simulink model "ControllerDesignModel_2023a"  (R2023a)
settings: Solver=FixedStepAuto  StartTime=0.0  StopTime=10  FixedStep=1/1000  RelTol=1e-3
values from neighbouring files (symbols this model uses):
  A = [-2.10   375 ... (first row only)    [ControllerDesign.m]
  B = [ 77 ... (first row only)    [ControllerDesign.m]
  C = [1 0 ... (first row only)    [ControllerDesign.m]
  D = [ 0 ... (first row only)    [ControllerDesign.m]
  IC = [0 deg2rad(30)]    [ControllerDesign.m]
  Kq = 0.17    [ControllerDesign.m]
libraries: simulink_extras x6, slctrlblks x2, slpidlib x1
settings Model: PacingRate=0.500000  Creator=EYEONIF  LastModifiedBy=AL-fa
settings DebuggingCC: AlgebraicLoopMsg=none
settings RTWCC: GPUComputeCapability=5.0

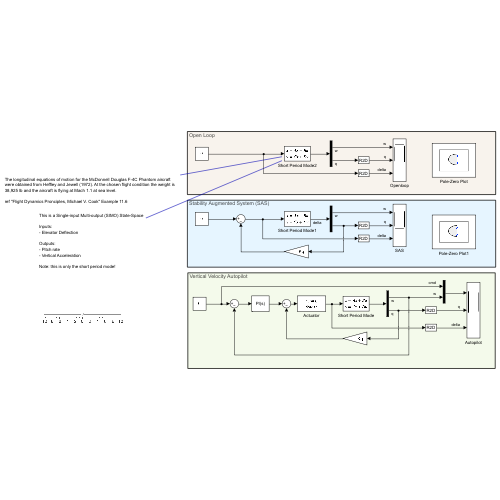
[thumbnail: Simulink's stored preview of the top-level diagram]
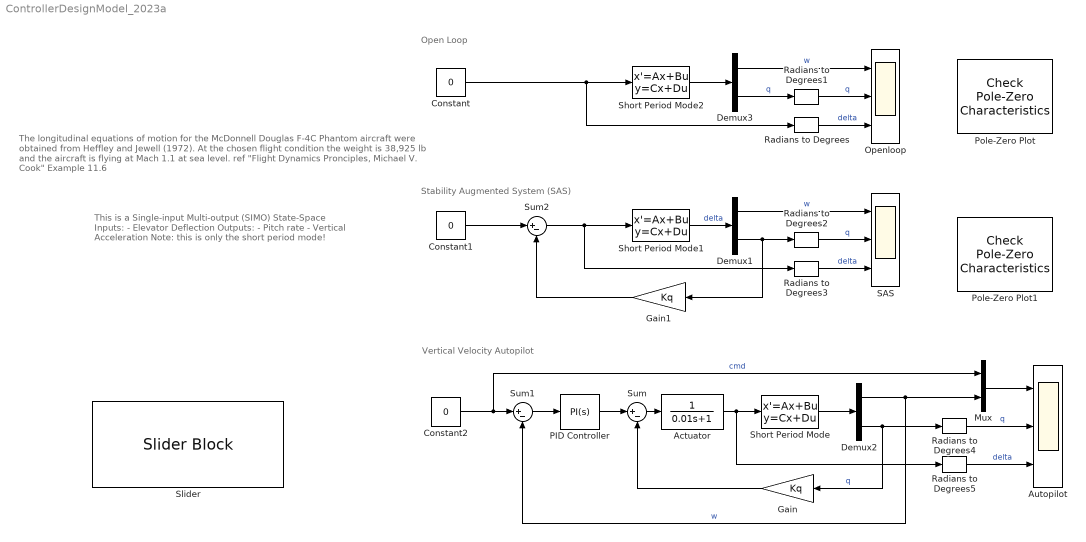
== system ControllerDesignModel_2023a ==
  note: Vertical Velocity Autopilot
  note: Stability Augmented System (SAS)
  note: Open Loop
  note: This is a Single-input Multi-output (SIMO) State-Space
      |
      | Inputs:
      | - Elevator Deflection
      |
      | Outputs:
      | - Pitch rate
      | - Vertical Acceleration
      |
      | Note: this is only the short period mode!
  note: The longitudinal equations of motion for the McDonnell Douglas F-4C Phantom aircraft were obtained from Heffley and Jewell (1972). At the chosen flight condition the weight is 38,925 lb and the aircraft is flying at Mach 1.1 at sea level.
      |
      | ref "Flight Dynamics Pronciples, Michael V. Cook" Example 11.6
  Actuator : TransferFcn  Denominator=[0.01 1]
  Autopilot : Scope  NumInputPorts=3
  Constant : Constant  Value=0
  Constant1 : Constant  Value=0
  Constant2 : Constant  Value=0
  Demux1 : Demux  Outputs=2
  Demux2 : Demux  Outputs=2
  Demux3 : Demux  Outputs=2
  Gain : Gain  Gain=Kq
  Gain1 : Gain  Gain=Kq
  Mux : Mux  Inputs=2
  Openloop : Scope  NumInputPorts=3
  PID Controller : slpidlib/PID Controller  Controller=PI  Form=Parallel  TimeDomain=Continuous-time  UseExternalTs=off  SampleTime=-1  IntegratorMethod=Forward Euler  FilterMethod=Forward Euler  ControllerParametersSource=internal  P=0.0033589459075444  I=0.0222004569710193  UseKiTs=off  D=-0.000626484444605212  N=3.41903099930503  UseFilter=on  TunerSelectOption=Transfer Function Based (PID Tuner App)  InitialConditionSource=internal  InitialConditionForIntegrator=0  InitialConditionForFilter=0  DifferentiatorICPrevScaledInput=0  ExternalReset=none  TrackingMode=off  Kt=1  LimitOutput=off  SatLimitsSource=internal  UpperSaturationLimit=inf  LowerSaturationLimit=-inf  LinearizeAsGain=on  AntiWindupMode=none  Kb=1  LimitIntegrator=off  UpperIntegratorSaturationLimit=inf  LowerIntegratorSaturationLimit=-inf  POutMin=[]  POutMax=[]  IOutMin=[]  IOutMax=[]  DOutMin=[]  DOutMax=[]  NOutMin=[]  NOutMax=[]  SumOutMin=[]  SumOutMax=[]  SaturationOutMin=[]  SaturationOutMax=[]  PParamMin=[]  PParamMax=[]  IParamMin=[]  IParamMax=[]  DParamMin=[]  DParamMax=[]  NParamMin=[]  NParamMax=[]  KbParamMin=[]  KbParamMax=[]  KtParamMin=[]  KtParamMax=[]  KbOutMin=[]  KbOutMax=[]  KtOutMin=[]  KtOutMax=[]  IntegratorOutMin=[]  IntegratorOutMax=[]  FilterOutMin=[]  FilterOutMax=[]  SumI1OutMin=[]  SumI1OutMax=[]  SumI2OutMin=[]  SumI2OutMax=[]  SumI3OutMin=[]  SumI3OutMax=[]  SumI4OutMin=[]  SumI4OutMax=[]  SumDOutMin=[]  SumDOutMax=[]  DifferentiatorOutMin=[]  DifferentiatorOutMax=[]  FilterDiffOutCoefMin=[]  FilterDiffOutCoefMax=[]  ReciprocalOutMin=[]  ReciprocalOutMax=[]  SumDenOutMin=[]  SumDenOutMax=[]  SumNumOutMin=[]  SumNumOutMax=[]  DivideOutMin=[]  DivideOutMax=[]  UdiffTsProdOutMin=[]  UdiffTsProdOutMax=[]  NTsProdOutMin=[]  NTsProdOutMax=[]  UintegralTsProdOutMin=[]  UintegralTsProdOutMax=[]  UngainTsProdOutMin=[]  UngainTsProdOutMax=[]  ClampingZeroOutDataTypeStr=Inherit: Inherit via back propagation  ClampingZeroOutMin=[]  ClampingZeroOutMax=[]  FilterDenConstantOutDataTypeStr=Inherit: Inherit via back propagation  FilterDenConstantOutMin=[]  FilterDenConstantOutMax=[]  PCopyOutDataTypeStr=Inherit: Inherit via back propagation  PCopyOutMin=[]  PCopyOutMax=[]  NCopyOutDataTypeStr=Inherit: Inherit via back propagation  NCopyOutMin=[]  NCopyOutMax=[]  IntegratorContinuousStateAttributes=''  IntegratorStateMustResolveToSignalObject=off  IntegratorRTWStateStorageClass=Auto  FilterContinuousStateAttributes=''  FilterStateMustResolveToSignalObject=off  FilterRTWStateStorageClass=Auto  ParallelPVariant=InternalParameters  IdealPVariant=Disabled  IVariant=InternalParameters  DVariant=Disabled  IntegratorVariant=Continuous  SatVariant=Disabled  AWVariant=Passthrough  PCopyVariant=Disabled  TRVariant=Disabled  FdbkBlocksVariant=Forward  IdealPFdbkVariant=Disabled  SatFdbkVariant=Disabled  DerivativeFilterVariant=Disabled  NVariant=Disabled  NCopyVariant=Disabled_SignalSpec  FilterICVariant=Disabled  IntegratorICVariant=InternalICs  ExternalResetVariant=Disabled  TRSumVariant=Passthrough  SumFdbkVariant=Disabled  SumVariant=Sum_PI  TsampFilterVariant=InternalTs  TsampNgainVariant=Passthrough  TsampIntegralVariant=Disabled_SignalSpec  ExternalSaturationOutDataTypeStr=Inherit: Same as second input
  Pole-Zero Plot : slctrlblks/Model Verification/Check Pole-Zero Characteristics  InstantiateOnLoad=on  SaveOperatingPoints=off  LinearizationIOs={'/Constant', 1, 'in', 'on', '';'/Demux3', 2, 'out', 'on', ''}  LinearizeAt=SnapshotTimes  SnapshotTimes=[0]  TriggerType=rising  SampleTime=auto  RateConversionMethod=zoh  PreWarpFreq=10  UseExactDelayModel=off  UseFullBlockNameLabels=off  UseBusSignalLabels=off  enabled=on  stopWhenAssertionFail=off  export=off  ViewDlgPos=[]  LaunchViewOnOpen=off  OpenViewOnLoad=off  FrequencyUnits=rad/s  MagnitudeUnits=dB  PhaseUnits=deg  TimeUnits=seconds  EnableSettlingTime=off  SettlingTime=[]  EnablePercentOvershoot=off  PercentOvershoot=[]  EnableDampingRatio=off  DampingRatio=[]  EnableNaturalFrequency=off  NaturalFrequencyBound=>=  NaturalFrequency=[]
      settings: LibrarySourceBlock=slctrlblks/Linear Analysis Plots/Pole-Zero Plot  SaveToWorkspace=on  SaveName=openLoop
  Pole-Zero Plot1 : slctrlblks/Model Verification/Check Pole-Zero Characteristics  InstantiateOnLoad=on  SaveOperatingPoints=off  LinearizationIOs={'/Constant1', 1, 'in', 'off', '';'/Demux1', 2, 'out', 'off', ''}  LinearizeAt=SnapshotTimes  SnapshotTimes=[0]  TriggerType=rising  SampleTime=auto  RateConversionMethod=zoh  PreWarpFreq=10  UseExactDelayModel=off  UseFullBlockNameLabels=off  UseBusSignalLabels=off  enabled=on  stopWhenAssertionFail=off  export=off  ViewDlgPos=[]  LaunchViewOnOpen=off  OpenViewOnLoad=off  FrequencyUnits=rad/s  MagnitudeUnits=dB  PhaseUnits=deg  TimeUnits=seconds  EnableSettlingTime=off  SettlingTime=[]  EnablePercentOvershoot=off  PercentOvershoot=[]  EnableDampingRatio=off  DampingRatio=[]  EnableNaturalFrequency=off  NaturalFrequencyBound=>=  NaturalFrequency=[]
      settings: LibrarySourceBlock=slctrlblks/Linear Analysis Plots/Pole-Zero Plot  SaveToWorkspace=on  SaveName=SAS
  Radians to Degrees{,1..5} (6 alike) : simulink_extras/Transformations/Radians to Degrees
  SAS : Scope  NumInputPorts=3
  Short Period Mode : StateSpace  A=A  B=B  C=C  D=D  InitialCondition=0
  Short Period Mode1 : StateSpace  A=A  B=B  C=C  D=D  InitialCondition=IC
  Short Period Mode2 : StateSpace  A=A  B=B  C=C  D=D  InitialCondition=IC
  Slider : SliderBlock  LabelPosition=Hide  ScaleMin=-10  ScaleMax=10
  Sum : Sum  Inputs=|+-
  Sum1 : Sum  Inputs=|+-
  Sum2 : Sum  Inputs=|+-
  wires:
  Short Period Mode/1 -> Demux2/1
  Demux2/1 -> Sum1/2, Mux/2  "w"
  Demux2/2 -> Radians to Degrees4/1, Gain/1  "q"
  Gain/1 -> Sum/2
  Constant2/1 -> Sum1/1, Mux/1  "cmd"
  Actuator/1 -> Radians to Degrees5/1, Short Period Mode/1
  Short Period Mode1/1 -> Demux1/1  "delta"
  Gain1/1 -> Sum2/2
  Sum2/1 -> Short Period Mode1/1, Radians to Degrees3/1
  Demux1/1 -> SAS/1  "w"
  Demux1/2 -> Gain1/1, Radians to Degrees2/1
  Demux3/2 -> Radians to Degrees1/1  "q"
  Short Period Mode2/1 -> Demux3/1
  Demux3/1 -> Openloop/1  "w"
  Constant/1 -> Radians to Degrees/1, Short Period Mode2/1
  Constant1/1 -> Sum2/1
  Mux/1 -> Autopilot/1
  Radians to Degrees/1 -> Openloop/3  "delta"
  Radians to Degrees1/1 -> Openloop/2  "q"
  Radians to Degrees2/1 -> SAS/2  "q"
  Radians to Degrees3/1 -> SAS/3  "delta"
  Radians to Degrees4/1 -> Autopilot/2  "q"
  Radians to Degrees5/1 -> Autopilot/3  "delta"
  Sum1/1 -> PID Controller/1
  PID Controller/1 -> Sum/1
  Sum/1 -> Actuator/1
